simulink model "Loader_Scanner_Model_Multi"  (R2025b)
settings: Solver=VariableStepDiscrete  StartTime=0.0  StopTime=144  RelTol=1e-3
model workspace (MAT data in the model file):
  check_toggle_ts = timeseries
  check_toggle_ts.Name = 'unnamed'
  check_toggle_ts.DataInfo = tsdata.datametadata
  check_toggle_ts.DataInfo.Interpolation = tsdata.interpolation
  check_toggle_ts.DataInfo.Interpolation.Fhandle : function handle (value not decoded)
  check_toggle_ts.DataInfo.Interpolation.Name = 'linear'
  check_toggle_ts.TimeInfo = tsdata.timemetadata
  check_toggle_ts.TimeInfo.Length = 144001
  check_toggle_ts.TimeInfo.DuplicateTimes = 0
  check_toggle_ts.TimeInfo.Time_ = [0 0.001 0.002 0.003 0.004 0.005 0.006 0.007 0.008 0.009 0.01 0.011 ... (144001 elements, 144001x1)]
  check_toggle_ts.TimeInfo.Initialized = 1
  check_toggle_ts.QualityInfo = tsdata.qualmetadata
  check_toggle_ts.Data_ = [0 0 0 0 0 0 0 0 0 0 0 0 ... (144001 elements, 144001x1)]
  courier_igt_hr = [8 9.99999999252e-07 1.999999 9.99999999252e-07 1.999999 9.99999999252e-07 1.999999 9.99999999252e-07 1.999999 1.00000000103e-06 1.999999 1.00000000103e-06 13.999999 9.99999997475e-07 1.999999 9.99999997475e-07 1.999999 9.99999997475e-07 1.999999 9.99999997475e-07 1.999999 9.99999997475e-07 1.999999 9.99999997475e-07 13.999999 9.99999997475e-07 1.999999 9.99999997475e-07 1.999999 9.99999997475e-07 1.999999 9.99999997475e-07 1.999999 9.99999997475e-07 1.999999 9.99999997475e-07 13.999999 9.99999997475e-07 1.999999 9.99999997475e-07 1.999999 9.99999997475e-07 1.999999 9.99999997475e-07 1.999999 9.99999997475e-07 1.999999 9.99999997475e-07 13.999999 9.99999997475e-07 1.999999 9.99999997475e-07 1.999999 9.99999997475e-07 1.999999 9.99999997475e-07 1.999999 9.99999997475e-07 1.999999 9.99999997475e-07 13.999999 9.99999997475e-07 1.999999 9.99999997475e-07 1.999999 9.99999997475e-07 1.999999 9.99999997475e-07 1.999999 9.99999997475e-07 1.999999 9.99999997475e-07]
  courier_transit_hr = 0.166666666667
  gate_times = [0; 8; 19.5; 32; 43.5; 56; 67.5; 80; 91.5; 104; 115.5; 124]
  gate_values = [0; 1; 0; 1; 0; 1; 0; 1; 0; 1; 0; 0]
  igt_hr = [6.12203823484; 0.203292095918; 1.00000000014e-06; 0.272568648048; 0.371684648953; 0.191636659489; 0.153134693822; 0.937426314749; 0.710664999117; 0.175073649204; 0.036845484859; 0.337726629294; 0.424636930437; 1.22407806268; 1.47033057458; 1.7539591026; 1.90849411566; 0.516521550415; 0.768166746317; 12.1795659695; 1.14750453149; 0.466667443837; 0.378596665848; 0.0257982091011; 0.214092181259; 1.83135491729; 9.99999997475e-07; 0.736543190445; 3.4048182897; 9.99999997475e-07; 0.314157643541; 0.61288260091; 0.0601477001856; 1.07595549042; 1.03000852215; 9.99999997475e-07; 0.756524512479; 0.186816664156; 0.228925132217; 11.5550102072; 0.385282050331; 0.10965527596; 0.618198070874; 1.18344533576; 0.0931398496331; 0.0131934287566; 0.223829802938; 3.06117936156; 0.668196188076; 1.32290740904; 1.3313454036; 3.8999232552; 10.5306563785; 0.122348378956; 9.99999997475e-07; 0.105263738994; 0.462627960178; 0.263698760986; 0.843924646266; 0.464961889929; 0.0542030164113; 0.633737063963; 0.489665395923; 5.06315208166; 1.52147925266; 1.67472818652; 1.96158155286; 9.99999997475e-07; 11.3378388666; 0.126307644344; 0.408113216537; 1.37063139177; 0.206248986786; 9.99999997475e-07; 0.490696896306; 0.241533850904; 0.514819858707; 9.99999997475e-07; 0.126000628469; 2.74321493568; 4.41723614363; 1.05222467986]
  igt_k = 1
  on_duty_ts = timeseries
  on_duty_ts.Name = 'unnamed'
  on_duty_ts.DataInfo = tsdata.datametadata
  on_duty_ts.DataInfo.Interpolation = tsdata.interpolation
  on_duty_ts.DataInfo.Interpolation.Fhandle : function handle (value not decoded)
  on_duty_ts.DataInfo.Interpolation.Name = 'linear'
  on_duty_ts.TimeInfo = tsdata.timemetadata
  on_duty_ts.TimeInfo.Length = 144001
  on_duty_ts.TimeInfo.DuplicateTimes = 0
  on_duty_ts.TimeInfo.Time_ = [0 0.001 0.002 0.003 0.004 0.005 0.006 0.007 0.008 0.009 0.01 0.011 ... (144001 elements, 144001x1)]
  on_duty_ts.TimeInfo.Initialized = 1
  on_duty_ts.QualityInfo = tsdata.qualmetadata
  on_duty_ts.Data_ = [0 0 0 0 0 0 0 0 0 0 0 0 ... (144001 elements, 144001x1)]
  psd_fixed = 0.333333333333
  psd_mu = -1.09861228867
  psd_sigma = 1.08921548281
  rack_entity_id = [1; 2; 3; 4; 5; 6; 7; 8; 9; 10; 11; 12; 13; 14; 15; 16; 17; 18; 19; 20; 21; 22; 23; 24; 25; 26; 27; 28; 29; 30; 31; 32; 33; 34; 35; 36; 37; 38; 39; 40; 41; 42; 43; 44; 45; 46; 47; 48; 49; 50; 51; 52; 53; 54; 55; 56; 57; 58; 59; 60; 61; 62; 63; 64; 65; 66; 67; 68; 69; 70; 71; 72; 73; 74; 75; 76; 77; 78; 79; 80; 81; 82]
  rack_num_cases = [9; 5; 1; 6; 8; 4; 5; 7; 7; 5; 2; 4; 6; 4; 5; 5; 5; 4; 4; 10; 11; 7; 4; 4; 7; 4; 1; 3; 5; 1; 4; 5; 2; 4; 3; 1; 3; 3; 2; 5; 9; 6; 5; 9; 5; 2; 6; 7; 2; 7; 4; 3; 5; 5; 1; 5; 8; 6; 10; 5; 2; 6; 4; 7; 5; 4; 6; 1; 9; 3; 6; 10; 3; 1; 5; 5; 3; 1; 2; 3; 5; 4]
  rack_slide_count = [20; 20; 20; 20; 20; 20; 20; 20; 20; 20; 20; 20; 20; 20; 20; 20; 20; 20; 16; 20; 20; 20; 20; 20; 20; 20; 20; 20; 20; 20; 20; 20; 20; 20; 20; 20; 20; 20; 6; 20; 20; 20; 20; 20; 20; 20; 20; 20; 20; 20; 20; 15; 20; 20; 20; 20; 20; 20; 20; 20; 20; 20; 20; 20; 20; 20; 20; 3; 20; 20; 20; 20; 20; 20; 20; 20; 20; 20; 20; 20; 20; 12]
  scanners_full = -1
  svc_times = [0; 8; 19.5]
  svc_values = [0; 1; 0]
values from neighbouring files (symbols this model uses):
  m = min(v)    [run_loader_scanner_model_multi_stress_v1_2_final_verified.m]    (also in run_slide_model_daily_scenarios_v2.m; run_slide_model_daily_scenarios_v2_scannerbank_v2.m)
  n = round(v(end))    [run_loader_scanner_model_multi_stress_v1_2_final_verified.m]    (also in run_slide_model_daily_scenarios_v2.m = numel(logs); run_slide_model_daily_scenarios_v2_scannerbank_v2.m)
  TestRack_IntergenerationTime = S(testIdx).rack_dt    [run_loader_scanner_model_multi_stress_v1_2_final_verified.m]
undefined symbols (not defined in the file or in its folder): entity, recordSlideCount
settings Model: Creator=bayes  LastModifiedBy=bayes

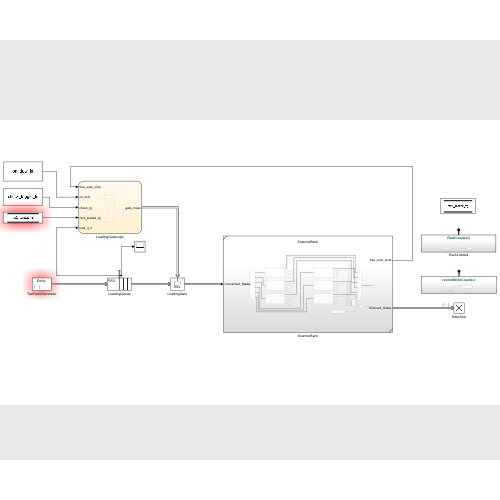
[thumbnail: Simulink's stored preview of the top-level diagram]
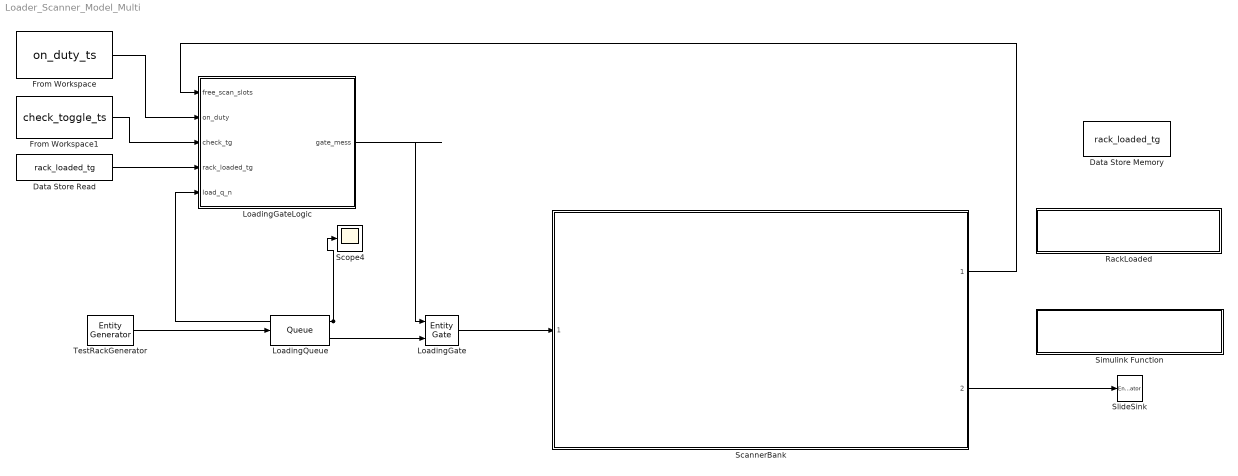
== system Loader_Scanner_Model_Multi ==
  Data Store Memory : DataStoreMemory  DataStoreName=rack_loaded_tg  WriteAfterWriteMsg=warning  ShowAdditionalParam=off  OutDataTypeStr=boolean
  Data Store Read : DataStoreRead  DataStoreName=rack_loaded_tg  IndexOptions=Index vector (dialog)  Indices=1  OutputSizes=1
  From Workspace : FromWorkspace  VariableName=on_duty_ts  OutDataTypeStr=boolean
  From Workspace1 : FromWorkspace  VariableName=check_toggle_ts  OutDataTypeStr=boolean
  LoadingGate : EntityGate  InputPortMessageModes=m,m  OutputPortMessageModes=m  OperatingMode=Release gate
  LoadingGateLogic : Stateflow chart  TreatAsAtomicUnit=on
  LoadingQueue : Queue  InputPortMessageModes=m  OutputPortMessageModes=n,m  Capacity=inf  NumberEntitiesInBlock=on
      settings: OutputPortMap=o1,o5
  RackLoaded : Subsystem  TreatAsAtomicUnit=on
  ScannerBank : Subsystem  ReferencedSubsystem=ScannerBank
  Scope4 : Scope
      settings: ActiveDisplayYMinimum=-507.99999999999989  ActiveDisplayYMaximum=4582  DataLoggingVariableName=ScopeData4
  Simulink Function : Subsystem  TreatAsAtomicUnit=on
  SlideSink : EntityTerminator  InputPortMessageModes=m  EntryAction=recordSlideCount(entity.SlideCount);
  TestRackGenerator : EntityGenerator  OutputPortMessageModes=m  Period=TestRack_IntergenerationTime  GenerateAction=entity.SlideCount = TestRack_SlideCount;  AttributeName=SlideCount  AttributeInitialValue=20  EntityType=Structured  EntityTypeName=Entity
  wires:
  LoadingGateLogic/1(gate_mess) -> LoadingGate/1
  LoadingQueue/2 -> LoadingGate/2
  TestRackGenerator/1 -> LoadingQueue/1
  LoadingQueue/1 -> LoadingGateLogic/5(load_q_n), Scope4/1
  From Workspace/1 -> LoadingGateLogic/2(on_duty)
  From Workspace1/1 -> LoadingGateLogic/3(check_tg)
  Data Store Read/1 -> LoadingGateLogic/4(rack_loaded_tg)
  LoadingGate/1 -> ScannerBank/1
  ScannerBank/1 -> LoadingGateLogic/1(free_scan_slots)
  ScannerBank/2 -> SlideSink/1

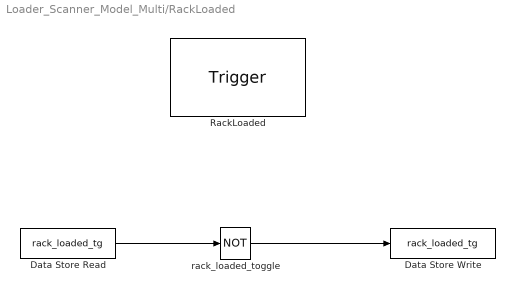
== system Loader_Scanner_Model_Multi/RackLoaded ==
  RackLoaded : TriggerPort  TriggerType=function-call  IsSimulinkFunction=on  FunctionName=RackLoaded  FunctionVisibility=scoped  VariantControl=(inherit)
  Data Store Read : DataStoreRead  DataStoreName=rack_loaded_tg  IndexOptions=Index vector (dialog)  Indices=1  OutputSizes=1
  Data Store Write : DataStoreWrite  DataStoreName=rack_loaded_tg  IndexOptions=Index vector (dialog)  Indices=1  OutputSizes=1
  rack_loaded_toggle : Logic  Operator=NOT  AllPortsSameDT=off  OutDataTypeStr=boolean
  wires:
  Data Store Read/1 -> rack_loaded_toggle/1
  rack_loaded_toggle/1 -> Data Store Write/1

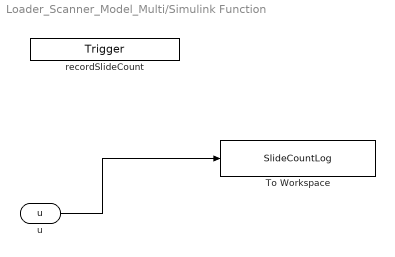
== system Loader_Scanner_Model_Multi/Simulink Function ==
  recordSlideCount : TriggerPort  TriggerType=function-call  IsSimulinkFunction=on  FunctionName=recordSlideCount  FunctionVisibility=scoped  VariantControl=(inherit)
  To Workspace : ToWorkspace  VariableName=SlideCountLog  SaveFormat=Timeseries  SampleTime=-1
  u : ArgIn  DisableCoverage=on  ArgumentName=u
  wires:
  u/1 -> To Workspace/1

== stateflow chart Loader_Scanner_Model_Multi/LoadingGateLogic ==
  state LOADING
    entry:
    last_rack_loaded_tg = rack_loaded_tg;
    gate_mess.data = 1;
    send(gate_mess);
  state LOAD
    entry:
    if racks_to_load < int32(0)
    if (load_q_n <= 0) || (free_scan_slots <= 0)
    racks_to_load = int32(0);
    elseif load_q_n < free_scan_slots
    racks_to_load = int32(load_q_n);
    else
    racks_to_load = int32(free_scan_slots);
    end
    end
  state OFF_DUTY
  state ON_DUTY
  state LOADING_COMPLETE
    entry:
    last_check_tg = check_tg;
    racks_to_load = int32(-1);
  LOADING -> LOAD : [rack_loaded_tg ~= last_rack_loaded_tg]/{racks_to_load = racks_to_load - int32(1);}
  LOAD -> LOADING [order 2] : [racks_to_load > int32(0)]
  OFF_DUTY -> LOAD : [on_duty]
  ON_DUTY -> LOAD [order 2] : [~on_duty]
  LOAD -> LOADING_COMPLETE [order 1] : [racks_to_load <= int32(0)]
  ON_DUTY -> LOAD [order 1] : [check_tg ~= last_check_tg]
  (default) -> OFF_DUTY
  LOADING_COMPLETE -> ON_DUTY [order 1] : [on_duty]
  LOADING_COMPLETE -> OFF_DUTY [order 2] : [~on_duty]
  data: free_scan_slots input double; on_duty input boolean; check_tg input boolean; rack_loaded_tg input boolean; gate_mess output; last_check_tg local boolean =0; load_q_n input double; last_rack_loaded_tg local boolean =0; racks_to_load local int32 =-1
